simulink model "dynamics_generate"  (R2022a)
settings: Solver=FixedStepAuto  StartTime=0.0  StopTime=100  FixedStep=0.1  RelTol=1e-3
values from neighbouring files (symbols this model uses):
  A = [0 0.3 0.4 0.3; 0.3 0 0.5 0; 0.4 0.5 0 0.3; 0.3 0 0.3 0]    [InitialInputsGenerate.m]    (also in initializer.m)
  b = [0.3 0.2 0.5 0.4]    [InitialInputsGenerate.m]    (also in initializer.m)
  c = [9.0 7.0 11.0 7.0]    [InitialInputsGenerate.m]    (also in initializer.m)
  dif = [1.0 1.0 1.0 1.0]    [InitialInputsGenerate.m]    (also in initializer.m = [1.0 1.0 1.0 10])
  get = [17.0 16.0 16.0 17.0]    [InitialInputsGenerate.m]    (also in initializer.m)
  h = [0 1 1 0]    [InitialInputsGenerate.m]    (also in initializer.m)
  x0 = [16.5 16.5 16.5 16.5]    [InitialInputsGenerate.m]    (also in initializer.m)
settings Model: Creator=Michael  LastModifiedBy=kimm58
settings RTWCC: GenCodeOnly=on

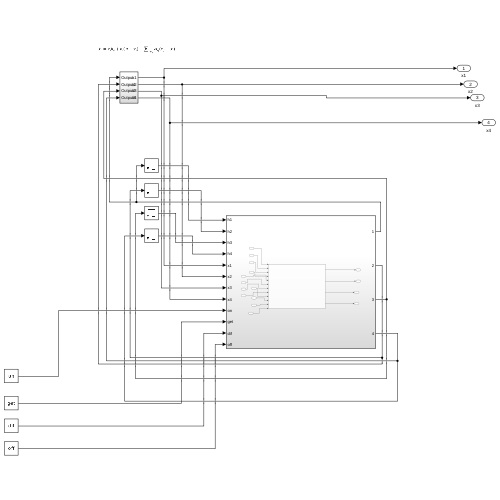
[thumbnail: Simulink's stored preview of the top-level diagram]
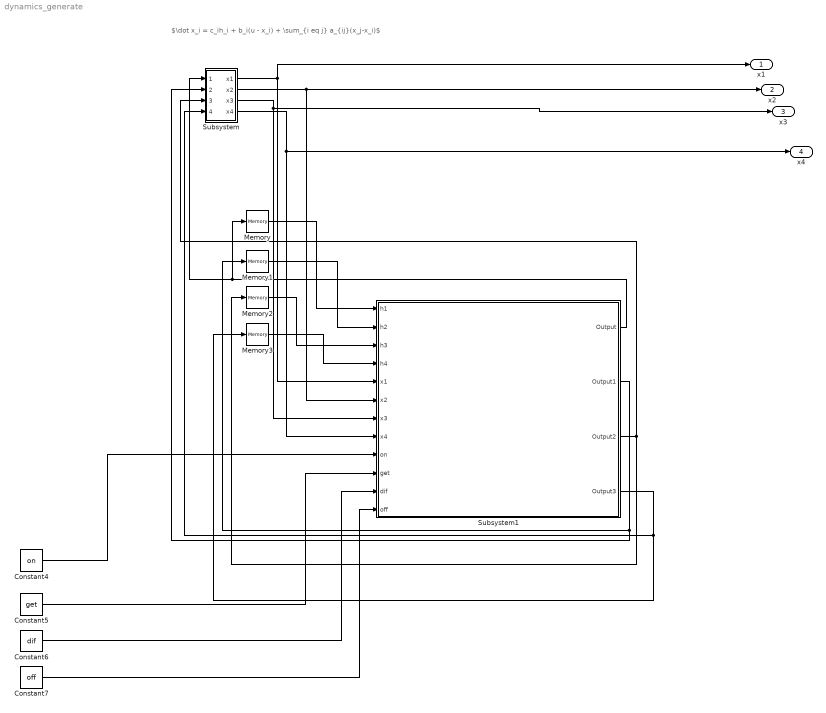
== system dynamics_generate ==
  note: $\dot x_i = c_ih_i + b_i(u - x_i) + \sum_{i\neq j} a_{ij}(x_j-x_i)$
  Constant4 : Constant  Value=on
  Constant5 : Constant  Value=get
  Constant6 : Constant  Value=dif
  Constant7 : Constant  Value=off
  Memory : Memory  InitialCondition=h(1)  InheritSampleTime=on
  Memory1 : Memory  InitialCondition=h(2)  InheritSampleTime=on
  Memory2 : Memory  InitialCondition=h(3)  InheritSampleTime=on
  Memory3 : Memory  InitialCondition=h(4)  InheritSampleTime=on
  Subsystem : Subsystem
  Subsystem1 : Subsystem
  x1 : Outport
  x2 : Outport  Port=2
  x3 : Outport  Port=3
  x4 : Outport  Port=4
  wires:
  Subsystem/1(x1) -> Subsystem1/5(x1), x1/1
  Subsystem/2(x2) -> x2/1, Subsystem1/6(x2)
  Subsystem/3(x3) -> x3/1, Subsystem1/7(x3)
  Subsystem/4(x4) -> x4/1, Subsystem1/8(x4)
  Constant5/1 -> Subsystem1/10(get)
  Constant7/1 -> Subsystem1/12(off)
  Memory2/1 -> Subsystem1/3("h3 ")
  Memory/1 -> Subsystem1/1("h1 ")
  Subsystem1/1(Output) -> Subsystem/1(Output), Memory/1
  Subsystem1/4(Output3) -> Subsystem/4(Output3), Memory3/1
  Subsystem1/3(Output2) -> Memory2/1, Subsystem/3(Output2)
  Constant4/1 -> Subsystem1/9(on)
  Memory1/1 -> Subsystem1/2("h2 ")
  Constant6/1 -> Subsystem1/11(dif)
  Memory3/1 -> Subsystem1/4(h4)
  Subsystem1/2(Output1) -> Subsystem/2(Output1), Memory1/1

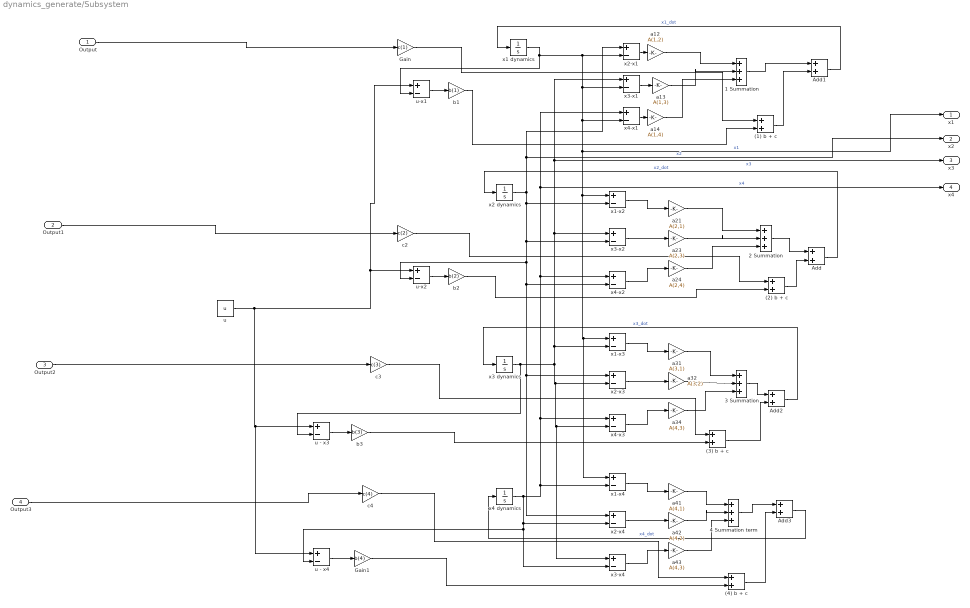
== system dynamics_generate/Subsystem ==
  Output : Inport
  Output1 : Inport  Port=2
  Output2 : Inport  Port=3
  Output3 : Inport  Port=4
  (1) b + c : Sum
  (2) b + c : Sum
  (3) b + c : Sum
  (4) b + c : Sum
  1 Summation : Sum  Inputs=++|+
  2 Summation : Sum  Inputs=++|+
  3 Summation : Sum  Inputs=++|+
  4 Summation term : Sum  Inputs=++|+
  Add{,1..3} (4 alike) : Sum
  Gain : Gain  Gain=c(1)
  Gain1 : Gain  Gain=b(4)
  a12 : Gain  Gain=A(1,2)
  a13 : Gain  Gain=A(1,3)
  a14 : Gain  Gain=A(1,4)
  a21 : Gain  Gain=A(2,1)
  a23 : Gain  Gain=A(2,3)
  a24 : Gain  Gain=A(2,4)
  a31 : Gain  Gain=A(3,1)
  a32 : Gain  Gain=A(3,2)
  a34 : Gain  Gain=A(4,3)
  a41 : Gain  Gain=A(4,1)
  a42 : Gain  Gain=A(4,2)
  a43 : Gain  Gain=A(4,3)
  b1 : Gain  Gain=b(1)
  b2 : Gain  Gain=b(2)
  b3 : Gain  Gain=b(3)
  c2 : Gain  Gain=c(2)
  c3 : Gain  Gain=c(3)
  c4 : Gain  Gain=c(4)
  u : Constant  Value=u
  u - x3 : Sum  Inputs=+-
  u - x4 : Sum  Inputs=+-
  u-x1 : Sum  Inputs=+-
  u-x2 : Sum  Inputs=+-
  x1 dynamics : Integrator  InitialCondition=x0(1)
  x1-x2 : Sum  Inputs=+-
  x1-x3 : Sum  Inputs=+-
  x1-x4 : Sum  Inputs=+-
  x2 dynamics : Integrator  InitialCondition=x0(2)
  x2-x1 : Sum  Inputs=+-
  x2-x3 : Sum  Inputs=+-
  x2-x4 : Sum  Inputs=+-
  x3 dynamics : Integrator  InitialCondition=x0(3)
  x3-x1 : Sum  Inputs=+-
  x3-x2 : Sum  Inputs=+-
  x3-x4 : Sum  Inputs=+-
  x4 dynamics : Integrator  InitialCondition=x0(4)
  x4-x1 : Sum  Inputs=+-
  x4-x2 : Sum  Inputs=+-
  x4-x3 : Sum  Inputs=+-
  x1 : Outport
  x2 : Outport  Port=2
  x3 : Outport  Port=3
  x4 : Outport  Port=4
  wires:
  Output2/1 -> c3/1
  (4) b + c/1 -> Add3/2
  a41/1 -> 4 Summation term/1
  u - x4/1 -> Gain1/1
  a42/1 -> 4 Summation term/2
  b2/1 -> (2) b + c/2
  b3/1 -> (3) b + c/2
  Output3/1 -> c4/1
  x2-x4/1 -> a42/1
  (3) b + c/1 -> Add2/2
  a31/1 -> 3 Summation/1
  a34/1 -> 3 Summation/3
  4 Summation term/1 -> Add3/1
  a12/1 -> 1 Summation/1
  u - x3/1 -> b3/1
  u-x2/1 -> b2/1
  x2-x1/1 -> a12/1
  Add/1 -> x2 dynamics/1  "x2_dot"
  a21/1 -> 2 Summation/1
  a32/1 -> 3 Summation/2
  x1-x4/1 -> a41/1
  Add1/1 -> x1 dynamics/1  "x1_dot"
  Add2/1 -> x3 dynamics/1  "x3_dot"
  x3-x1/1 -> a13/1
  Output/1 -> Gain/1
  u-x1/1 -> b1/1
  1 Summation/1 -> Add1/1
  x1-x2/1 -> a21/1
  c2/1 -> (2) b + c/1
  b1/1 -> (1) b + c/2
  a24/1 -> 2 Summation/3
  3 Summation/1 -> Add2/1
  (1) b + c/1 -> Add1/2
  Output1/1 -> c2/1
  x1-x3/1 -> a31/1
  x4-x2/1 -> a24/1
  2 Summation/1 -> Add/1
  u/1 -> u - x4/1, u - x3/1, u-x1/1, u-x2/1
  a23/1 -> 2 Summation/2
  a14/1 -> 1 Summation/3
  c4/1 -> (4) b + c/1
  x3-x2/1 -> a23/1
  a43/1 -> 4 Summation term/3
  c3/1 -> (3) b + c/1
  x4 dynamics/1 -> x3-x4/2, u - x4/2, x2-x4/2, x4-x1/1, x4/1, x4-x2/1, x4-x3/1, x1-x4/2  "x4"
  x3-x4/1 -> a43/1
  x4-x1/1 -> a14/1
  x2 dynamics/1 -> x2/1, x2-x1/1, x3-x2/2, x2-x4/1, x2-x3/1, x4-x2/2, u-x2/2, x1-x2/2  "x2"
  x1 dynamics/1 -> u-x1/2, x1-x4/1, x1-x3/1, x1-x2/1, x1/1, x4-x1/2, x3-x1/2, x2-x1/2  "x1"
  x2-x3/1 -> a32/1
  Add3/1 -> x4 dynamics/1  "x4_dot"
  x4-x3/1 -> a34/1
  Gain1/1 -> (4) b + c/2
  (2) b + c/1 -> Add/2
  x3 dynamics/1 -> u - x3/2, x3-x4/1, x4-x3/2, x2-x3/2, x1-x3/2, x3/1, x3-x1/1, x3-x2/1  "x3"
  a13/1 -> 1 Summation/2
  Gain/1 -> (1) b + c/1

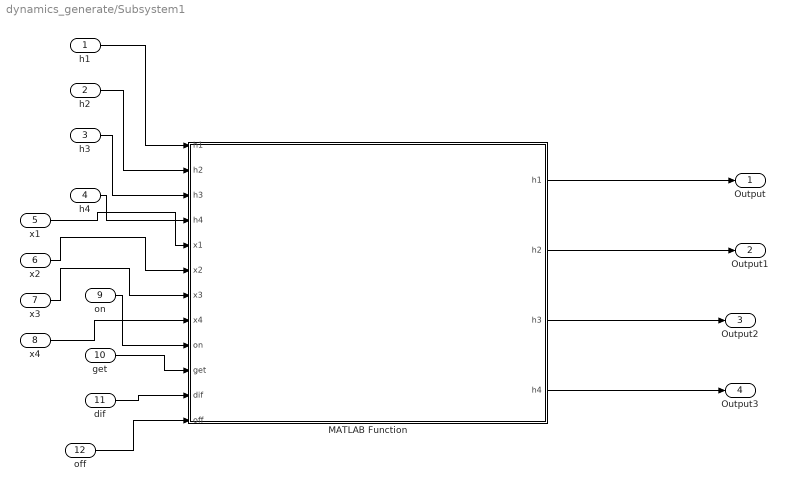
== system dynamics_generate/Subsystem1 ==
  "h1 " : Inport
  "h2 " : Inport  Port=2
  "h3 " : Inport  Port=3
  h4 : Inport  Port=4
  x1 : Inport  Port=5
  x2 : Inport  Port=6
  x3 : Inport  Port=7
  x4 : Inport  Port=8
  on : Inport  Port=9
  get : Inport  Port=10
  dif : Inport  Port=11
  off : Inport  Port=12
  MATLAB Function : MATLAB Function  TreatAsAtomicUnit=on
  Output : Outport
  Output1 : Outport  Port=2
  Output2 : Outport  Port=3
  Output3 : Outport  Port=4
  wires:
  MATLAB Function/2(h2) -> Output1/1
  MATLAB Function/3(h3) -> Output2/1
  MATLAB Function/4(h4) -> Output3/1
  MATLAB Function/1(h1) -> Output/1
  "h1 "/1 -> MATLAB Function/1("h1 ")
  "h2 "/1 -> MATLAB Function/2("h2 ")
  "h3 "/1 -> MATLAB Function/3("h3 ")
  x1/1 -> MATLAB Function/5(x1)
  x2/1 -> MATLAB Function/6(x2)
  h4/1 -> MATLAB Function/4("h4 ")
  x3/1 -> MATLAB Function/7(x3)
  x4/1 -> MATLAB Function/8(x4)
  on/1 -> MATLAB Function/9(on)
  get/1 -> MATLAB Function/10(get)
  dif/1 -> MATLAB Function/11(dif)
  off/1 -> MATLAB Function/12(off)

== matlab function dynamics_generate/Subsystem1/MATLAB Function ==
  settings: updateMethod=DISCRETE
  data: h1 input; h1 output; h2 input; h3 input; h4 input; x1 input; x2 input; x3 input; x4 input; on input; get input; dif input; off input; h2 output; h3 output; h4 output
function [h1,h2,h3,h4] = SelectHeaters(h1,h2,h3,h4,x1,x2,x3,x4,on,get,dif,off)
x = [x1,x2,x3,x4];
h = [h1,h2,h3,h4];
persistent locations;
hnew = zeros(1,4);
if isempty(locations)
    locations = h;
end
ind = find(locations == 1);

biggestdiff = 0;
newind = ind;

for i = 1:1:4
    if x(i) <= get(i) && x(ind(1)) - x(i) >= dif(i)
        curdiff = on(i)-x(i);
        if curdiff > biggestdiff
            biggestdiff = curdiff;
            newind(1) = i;
        end
    end
end

locations(newind(1)) = 1;
if x(newind(1)) <= on(newind(1)) && x(newind(1)) < off(newind(1))
    hnew(newind(1)) = 1;
end

biggestdiff = 0;

for i = 1:1:4
    if x(i) <= get(i) && x(ind(1)) - x(i) >= dif(i) && i ~= newind(1)
        curdiff = on(i)-x(i);
        if curdiff > biggestdiff
            biggestdiff = curdiff;
            newind(2) = i;
        end
    end
end

locations(newind(2)) = 1;
if x(newind(2)) <= on(newind(2)) && x(newind(2)) < off(newind(2))
    hnew(newind(2)) = 1;
end

h1 = hnew(1);
h2 = hnew(2);
h3 = hnew(3);
h4 = hnew(4);
